simulink model "pendulo"  (R2015a)
settings: Solver=ode3  StartTime=0.0  StopTime=simtime  FixedStep=0.001  RelTol=1e-2
values from neighbouring files (symbols this model uses):
  g = 9.8    [primeirolab.m]
  l = 0.5    [primeirolab.m]
  m = 1    [primeirolab.m]
  p1_0 = (1/6)*m*l*l*(8*dteta1+3*dteta2*cos(teta1_0-teta2_0))    [primeirolab.m]
  p2_0 = (1/6)*m*l*l*(2*dteta2+3*dteta1*cos(teta1_0-teta2_0))    [primeirolab.m]
  teta1_0 = atan2(x1,y1)    [primeirolab.m]
  teta2_0 = atan2(x-x1,y-y1)    [primeirolab.m]
settings Model: Creator=abran  LastModifiedBy=abran

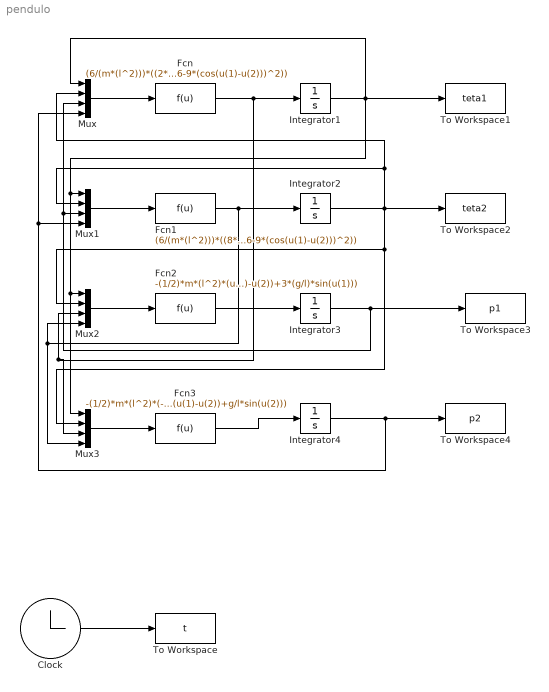
== system pendulo ==
  Clock : Clock
  Fcn : Fcn  Expr=(6/(m*(l^2)))*((2*u(3)-3*cos(u(1)-u(2))*u(4))/(16-9*(cos(u(1)-u(2)))^2))
  Fcn1 : Fcn  Expr=(6/(m*(l^2)))*((8*u(4)-3*cos(u(1)-u(2))*u(3))/(16-9*(cos(u(1)-u(2)))^2))
  Fcn2 : Fcn  Expr=-(1/2)*m*(l^2)*(u(3)*u(4)*sin(u(1)-u(2))+3*(g/l)*sin(u(1)))
  Fcn3 : Fcn  Expr=-(1/2)*m*(l^2)*(-u(3)*u(4)*sin(u(1)-u(2))+g/l*sin(u(2)))
  Integrator1 : Integrator  InitialCondition=teta1_0
  Integrator2 : Integrator  InitialCondition=teta2_0
  Integrator3 : Integrator  InitialCondition=p1_0
  Integrator4 : Integrator  InitialCondition=p2_0
  Mux{,1..3} (4 alike) : Mux
  To Workspace : ToWorkspace  VariableName=t  SampleTime=-1
      settings: MaxDataPoints=2500001
  To Workspace1 : ToWorkspace  VariableName=teta1  SampleTime=-1
  To Workspace2 : ToWorkspace  VariableName=teta2  SampleTime=-1
  To Workspace3 : ToWorkspace  VariableName=p1  SampleTime=-1
  To Workspace4 : ToWorkspace  VariableName=p2  SampleTime=-1
  wires:
  Integrator1/1 -> Mux2/1, Mux3/1, Mux1/1, Mux/1, To Workspace1/1
  Integrator2/1 -> Mux3/2, Mux2/2, Mux1/2, Mux/2, To Workspace2/1
  Integrator3/1 -> Mux1/3, Mux/3, To Workspace3/1
  Integrator4/1 -> Mux1/4, Mux/4, To Workspace4/1
  Fcn/1 -> Mux3/3, Mux2/3, Integrator1/1
  Fcn1/1 -> Mux3/4, Mux2/4, Integrator2/1
  Fcn2/1 -> Integrator3/1
  Fcn3/1 -> Integrator4/1
  Mux/1 -> Fcn/1
  Mux3/1 -> Fcn3/1
  Mux2/1 -> Fcn2/1
  Mux1/1 -> Fcn1/1
  Clock/1 -> To Workspace/1
